simulink model "MCU_speedcontrol_dsPIC33AK128MC106_MCLV_48V_300W_2022A"  (R2022a)
settings: Solver=FixedStepDiscrete  StartTime=0.0  StopTime=10.0  FixedStep=50e-6  RelTol=1e-3  EnableMultiTasking=on
undefined symbols (not defined in the file or in its folder): A0, A4, ADC, B0, C10, C11, C6, C7, C8, control, D11, D12, DiscIntNeverNeededParam, inverter, Max, MaxPer, motor, ms, NumBits1, NumBits2, P1, P17, P20, P39, P40, P41, P43, P44, P60, P61, Pin, PosRange1, PosRange2, PWM1_Trg1, Resol, s, Slope1, Slope2, us
libraries: simulink x31, MCHP_Blockset x19
(part 1 of 5)
settings Model: ExtModeEnableFloating=off  ExtModeTrigDuration=20  Creator=rdelpoux  LastModifiedBy=rdelpoux
settings SolverCC: AlgebraicLoopSolver=TrustRegion
settings OptimizationCC: DefaultParameterBehavior=Inlined  DefaultUnderspecifiedDataType=single  InlineInvariantSignals=on  EnhancedBackFolding=on  BooleansAsBitfields=on  PassReuseOutputArgsAs=Individual arguments  ZeroExternalMemoryAtStartup=off  ZeroInternalMemoryAtStartup=off  OptimizeBlockOrder=speed  DifferentSizesBufferReuse=on  EfficientTunableParamExpr=on
settings DebuggingCC: MultiTaskDSMMsg=none  MultiTaskCondExecSysMsg=none  MultiTaskRateTransMsg=warning  ParameterTunabilityLossMsg=error  ArithmeticOperatorsInVariantConditions=warning
settings HardwareCC: ProdBitPerPointer=32  ProdBitPerSizeT=32  ProdBitPerPtrDiffT=32  ProdLargestAtomicInteger=Long  ProdWordSize=32  ProdLongLongMode=on  ProdHWDeviceType=Generic->Custom
settings ModelReferenceCC: EnableRefExpFcnMdlSchedulingChecks=off  ModelReferenceNumInstancesAllowed=Single
settings SFSimCC: MATLABDynamicMemAlloc=off  CustomCodeUndefinedFunction=UseInterfaceOnly
settings RTWCC: Description=Microchip Embedded Target dsPIC33A (real-time)  SystemTargetFile=MCHP_dsPIC33A_stf.tlc  TLCOptions="-aExtModeXCPClassicInterface=0  -aCreateExtModeTypes=1 -aExtModeXCPSimulationTimeInTicks=1"  TemplateMakefile=MCHP_dsPIC33A.tmf
settings CodeAppCC: ForceParamTrailComments=on  IgnoreCustomStorageClasses=off  MaxIdLength=255  OperatorAnnotations=on  SimulinkDataObjDesc=on  SFDataObjDesc=on  InsertBlockDesc=on
settings STFCustomTargetCC: TargetLibSuffix=_lib.a  TargetLangStandard=C99 (ISO)  MultiwordLength=256  CombineOutputUpdateFcns=on  CombineSignalStateStructs=on  SuppressErrorStatus=on  ERTCustomFileBanners=on  SupportContinuousTime=off  RemoveResetFunc=on  MATLABClassNameForMDSCustomization=Simulink.SoftwareTarget.ERTCustomization  GRTInterface=off  SystemTargetFile=MCHP_dsPIC33A_stf.tlc
settings ERTTargetCC: TargetLibSuffix=_lib.a  TargetLangStandard=C99 (ISO)  ParMdlRefBuildCompliant=off  CompOptLevelCompliant=off  ConcurrentExecutionCompliant=off  CombineSignalStateStructs=on  SuppressErrorStatus=on  SupportNonInlinedSFcns=on  ModelStepFunctionPrototypeControlCompliant=off  CPPClassGenCompliant=off  UseToolchainInfoCompliant=off  ExtModeTransport=1  ExtModeStaticAlloc=on  ExtModeStaticAllocSize=2048  ExtModeMexFile=ext_xcp  ExtModeIntrfLevel=Level2 - Open  InlinedParameterPlacement=NonHierarchical  ERTSrcFileBannerTemplate=MCHP_dsPIC_code_template.cgt  ERTHdrFileBannerTemplate=MCHP_dsPIC_code_template.cgt  ERTDataSrcFileTemplate=MCHP_dsPIC_code_template.cgt  ERTDataHdrFileTemplate=MCHP_dsPIC_code_template.cgt  ERTCustomFileTemplate=MCHP_main.tlc  MaxLineWidth=110

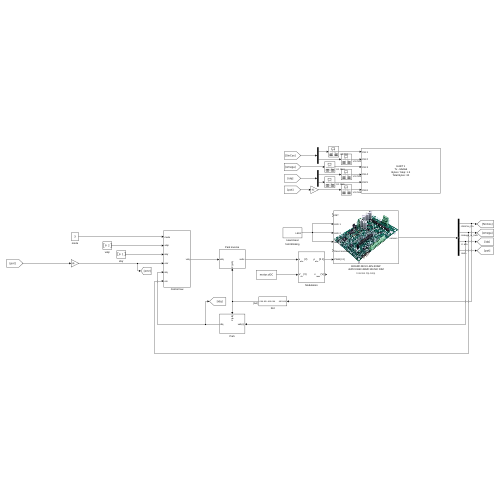
[thumbnail: Simulink's stored preview of the top-level diagram]
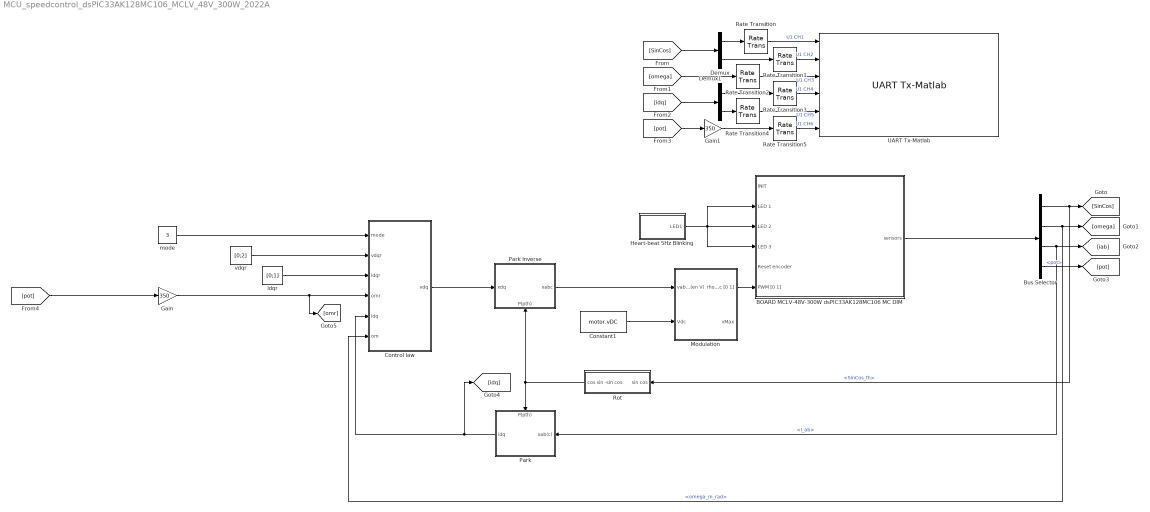
== system MCU_speedcontrol_dsPIC33AK128MC106_MCLV_48V_300W_2022A ==
  BOARD MCLV-48V-300W dsPIC33AK128MC106 MC DIM : Subsystem  mask(MCLV-48V-300W - dsPIC33AK128MC106 MC DIM){boardVariants=Internal Op-Amp, n=4, QEIResolution=4000, Switching_Frequency=20000, DeadTime=1e-6, QEI_Reset=on index signal, QEI_Offset_settings=0, QEIOffset=0}
      mask prompts: boardVariants "Board Variants"; n "Motor Pole Pairs"; QEIResolution "Optical Encoder Resolution Per Mechanical Rotation (lines)"; Switching_Frequency "PWM Switching Frequency (Hz)"; DeadTime "Dead Time (s)"; QEI_Reset "Optical encoder reset"; QEI_Offset_settings "Optical encoder offset (mechanical in rad)"; QEIOffset "Optical encoder offset (mechanical in rad)"
      mask help:
      | Template for creating Motor Control Algorithm using Microchip's MCLV-48V-300W Development Board and dsPIC33AK128MC106 Motor Control DIM.
      |
      | Template outputs:
      |   - Phase Currents (Ia and Ib)
      |   - DC Bus voltage and Bus current
      |   - Potentiometer
      |   - Push Buttons (0 when pressed, 1 for Btn 3 unconnected)
      |   - QEI Position and Velocity
      |   - MCU load and overload
      |
      | Template inputs:
      |   - INIT signal to trigger phase current offset measurement
      |   - LEDs
      |   - Reset encoder signal can be used to reset the encoder counter
      |   - PWM Duty cycle ratio [0 1]
      |
      | Note:
      | By default model and the template is configured to operate with fixed step-size of 50us.
      | This fixed step-size is synchronized with the PWM switching frequency and ADC conversion.
      |
      | Open subsystem (ctrl-u) for further customization.
      |
      | Warning:
      | Default configurations of the template are tested using the Microchip's Development Boards.
      | Any customization of the peripheral configurations needs to be verified with respect to device datasheet, hardware user guide and intended functionality.
      mask init:
      | BlksQEI = find_system(gcb,'FollowLinks','on','LookUnderMasks','all','ReferenceBlock','MCHP_Blockset/QEI/QEI');
      | QEI_Reset = get_param(gcb,'QEI_Reset');
      | if numel(BlksQEI) >= 1
      |     switch QEI_Reset
      |         case 'on index signal'
      |             set_param(BlksQEI{1},'PIMOD_mode','RESET position on each INDEX event');
      |         case 'on logical input (software)'        
      |             set_param(BlksQEI{1},'PIMOD_mode','position is cyclique between user defined boundaries'); 
      |         case 'custom setting'
      |             % do nothing 
      |     end
      | end % if
      | 
      |     BlksOpAmp = find_system(gcb,'FollowLinks','on','IncludeCommented','on','LookUnderMasks','all','ReferenceBlock','MCHP_Blockset/Analog IO/Op-Amp');
      |     if numel(BlksOpAmp) >= 1
      |         boardVariants = get_param(gcb,'boardVariants');
      |         switch boardVariants
      |             case 'internal Op-Amp'
      |                 set_param(BlksOpAmp{1},'Commented','off');
      |             case 'external Op-Amp'
      |                 set_param(BlksOpAmp{1},'Commented','on');
      |         end
      |     end % if
      settings: AttributesFormatString=%<boardVariants>
      mask Help: https://forum.microchip.com/s/sub-forums?&subForumId=a553l000000J2rNAAS&forumId=a553l000000J2pvAAC&subForumName=MATLAB&forumName=Development%20Tools&page=1&offset=0
      mask TypeOptions boardVariants: Internal Op-Amp | External Op-Amp
      mask TypeOptions QEI_Reset: on index signal | on logical input (software) | custom setting
      mask Callback QEI_Reset:
      | QEI_Reset = get_param(gcb,'QEI_Reset');
      | switch QEI_Reset
      |     case 'on index signal'
      |         QEIOffset = MCHP_Fun.Evalin('base','QEIOffset');
      |         set_param(gcb,'QEIOffset',num2str(QEIOffset));
      |         set_param(gcb,'MaskVisibilities',{'on';'on';'on';'on';'on';'on';'off';'on'});
      |     case 'on logical input (software)'
      |         set_param(gcb,'QEIOffset','0');
      |         set_param(gcb,'MaskVisibilities',{'on';'on';'on';'on';'on';'on';'off';'off'});
      |     case 'custom setting'
      |         set_param(gcb,'MaskVisibilities',{'on';'on';'on';'on';'on';'on';'off';'on'});
      |         % do nothing
      | end
      mask DialogControl boardParameters Prompt: Board
      mask DialogControl MotorParameters Prompt: Motor
      mask DialogControl n Tooltip: Number of pole pairs of the motor
      mask DialogControl QEIResolution Tooltip: encoder resolution per mechanical rotation
      mask DialogControl PWMParameters Prompt: PWM
      mask DialogControl QEIParameters Prompt: QEI
      mask DialogControl QEI_Reset Tooltip: enable encoder index signal if available. Otherwise align motor by applying a tension and set the rst input to 1
      mask DialogControl QEI_Offset_settings Tooltip: offset angle between encoder index and motor winding reference axis applied on theta_m and theta_e
      mask Display: image('MCHP_i_Board_MCLV_300W48V_reduced.jpg');
  Bus Selector : BusSelector  OutputSignals=optical coder.elec.SinCos_th,optical coder.mecc.omega_m_rad,ADC.I_ab,ADC.pot
  Constant1 : Constant  Value=motor.vDC  OutDataTypeStr=single
  Control law : Subsystem
  Demux : Demux  Outputs=2
  Demux1 : Demux  Outputs=2
  Gain : Gain  Gain=350
  Gain1 : Gain  Gain=350
  Heart-beat 5Hz Blinking : Subsystem
  Modulation : Subsystem  mask{modulation=Space Vector, mod=0}
      mask init:
      | switch modulation
      |     case 'Sinusoidale'
      |         mod = 0;
      |     otherwise
      |         mod = 1;
      | end
      mask TypeOptions modulation: Sinusoidale | Space Vector
      mask DialogControl DescGroupVar Prompt: Modulation interssecticve
      mask DialogControl DescTextVar Prompt: Choose between sinus or space vector modulation
      mask Display:
      | port_label('output', 1, '\rho_{abc} [0 1]', 'texmode','on')
      | port_label('output', 2, 'v_{\rm max} (V)', 'texmode','on')
      | port_label('input', 1, 'v_{abc} (V)', 'texmode','on')
      | port_label('input', 2, 'V_{dc} (V)', 'texmode','on')
  Park : Subsystem
      settings: PortSchema="{\"entries\":[{\"content\":{\"sides\":[{\"content\":{\"connectorIds\":[\"In1\"]},\"type\":\"ConnectorPlacement.EquallySpacedRectSide\",\"uuid\":\"ebf2fcb8-f94c-4630-a735-fb74e68b604e\"},{\"content\":{\"connectorIds\":[\"Out1\"],\"side\":\"RIGHT\"},\"type\":\"ConnectorPlacement.EquallySpacedRectSide\",\"uuid\":\"fb89ad3f-9420-4065-992c-c6d77ce245e0\"},{\"content\":{\"connectorIds\":[\"In2\"],\"side\":\"TOP\"},\"type\":\"ConnectorPlacement.EquallySpacedRectSide\",\"uuid\":\"0249ceba-2241-48c9-87d4-d9d6f381f2d7\"}]},\"type\":\"ConnectorPlacement.EquallySpacedConnector\",\"uuid\":\"eecfd82d-5918-403e-a677-09fe1d8cc737\"}],\"packageUris\":[\"http://schema.mathworks.com/mf0/Connector/R2020b\"],\"version\":\"1.0\"}"
  Park inverse : Subsystem
      settings: PortSchema="{\"entries\":[{\"content\":{\"sides\":[{\"content\":{\"connectorIds\":[\"In1\"]},\"type\":\"ConnectorPlacement.EquallySpacedRectSide\",\"uuid\":\"4c11ef0a-1978-4a73-9b5c-4d5650fcee33\"},{\"content\":{\"connectorIds\":[\"Out1\"],\"side\":\"RIGHT\"},\"type\":\"ConnectorPlacement.EquallySpacedRectSide\",\"uuid\":\"28284572-70c7-45ef-9db5-4b5788e96454\"},{\"content\":{\"side\":\"TOP\"},\"type\":\"ConnectorPlacement.EquallySpacedRectSide\",\"uuid\":\"3a1fbce2-0868-491b-8e3a-2b3a7a0d615d\"},{\"content\":{\"connectorIds\":[\"In2\"],\"side\":\"BOTTOM\"},\"type\":\"ConnectorPlacement.EquallySpacedRectSide\",\"uuid\":\"e63426ef-821a-4774-a922-a3f70d9b2116\"}]},\"type\":\"ConnectorPlacement.EquallySpacedConnector\",\"uuid\":\"285593a5-8af6-47f2-83d9-d6ebce98de71\"}],\"packageUris\":[\"http://schema.mathworks.com/mf0/Connector/R2020b\"],\"version\":\"1.0\"}"
  Rate Transition{,1..5} (6 alike) : RateTransition
  Rot : Subsystem
  UART Tx-Matlab : MCHP_Blockset/BUS UART/UART Tx-Matlab  UART_REF=1  CHANNELS=[1:6]  AllOrNothing=off  SampleTime=1e-3  MCHP_MASTERLINK=MCU_speedcontrol_dsPIC33AK128MC106_MCLV_48V_300W_2022A/BOARD MCLV-48V-300W dsPIC33AK128MC106 MC DIM/Microchip Master  MCHP_COMPILED_INFO="CompiledSampleTime= [0.0010000000000000000208   0 ];CompiledInportDataTypes=[  1   1   1   1   1   1 ];CompiledInportDataWidth=[1  1  1  1  1  1];"
      settings: SourceProductName=MPLAB Device Blocks for Simulink
  idqr : Constant  Value=[0;1]  OutDataTypeStr=single
  mode : Constant  Value=3  OutDataTypeStr=single
  vdqr : Constant  Value=[0;2]  OutDataTypeStr=single
  wires:
  BOARD MCLV-48V-300W dsPIC33AK128MC106 MC DIM/1(sensors) -> Bus Selector/1
  Bus Selector/1 -> Rot/1(sin cos), [SinCos]  "<SinCos_th>"
  Bus Selector/2 -> Control law/6(om), [omega]  "<omega_m_rad>"
  Bus Selector/3 -> Park/1(xab(c)), [iab]  "<I_ab>"
  Bus Selector/4 -> [pot]  "<pot>"
  Demux/1 -> Rate Transition/1
  Demux/2 -> Rate Transition1/1
  Demux1/1 -> Rate Transition3/1
  Demux1/2 -> Rate Transition4/1
  [pot] -> Gain1/1
  [idq] -> Demux1/1
  [omega] -> Rate Transition2/1
  [SinCos] -> Demux/1
  Rate Transition/1 -> UART Tx-Matlab/1  "U1 CH1"
  Rate Transition1/1 -> UART Tx-Matlab/2  "U1 CH2"
  Rate Transition2/1 -> UART Tx-Matlab/3  "U1 CH3"
  Rate Transition3/1 -> UART Tx-Matlab/4  "U1 CH4"
  Rate Transition4/1 -> UART Tx-Matlab/5  "U1 CH5"
  Rate Transition5/1 -> UART Tx-Matlab/6  "U1 CH6"
  Heart-beat 5Hz Blinking/1(LED1) -> BOARD MCLV-48V-300W dsPIC33AK128MC106 MC DIM/3(LED 2), BOARD MCLV-48V-300W dsPIC33AK128MC106 MC DIM/4(LED 3), BOARD MCLV-48V-300W dsPIC33AK128MC106 MC DIM/2(LED 1)
  Park inverse/1(xabc) -> Modulation/1("vabc (en V) ")
  Rot/1("cos sin -sin cos ") -> Park/2(P(pth)), Park inverse/2(P(pth))
  Constant1/1 -> Modulation/2(Vdc)
  Modulation/1(rho_abc [0 1]) -> BOARD MCLV-48V-300W dsPIC33AK128MC106 MC DIM/6(PWM [0 1])
  Park/1(idq) -> Control law/5(idq), [idq]
  idqr/1 -> Control law/3(idqr)
  vdqr/1 -> Control law/2(vdqr)
  mode/1 -> Control law/1(mode)
  [pot] -> Gain/1
  Control law/1(vdq) -> Park inverse/1(xdq)
  Gain/1 -> Control law/4(omr), [omr]
  Gain1/1 -> Rate Transition5/1
